simulink model "model_p3"  (R2020b)
settings: Solver=VariableStepAuto  StartTime=0.0  StopTime=10.0  RelTol=1e-3
settings Model: Creator=ADMIN  LastModifiedBy=ADMIN

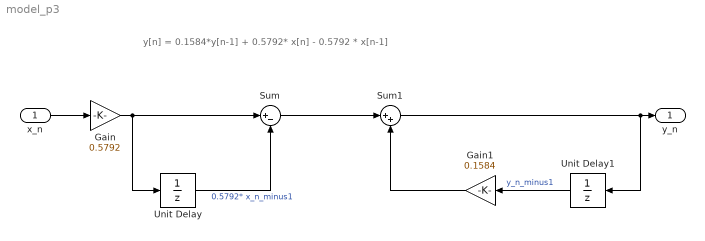
== system model_p3 ==
  note: y[n] = 0.1584*y[n-1] + 0.5792* x[n] - 0.5792 * x[n-1]
  x_n : Inport
  Gain : Gain  Gain=0.5792
  Gain1 : Gain  Gain=0.1584
  Sum : Sum  Inputs=|+-
  Sum1 : Sum  Inputs=|++
  Unit Delay : UnitDelay  SampleTime=-1  HasFrameUpgradeWarning=on
  Unit Delay1 : UnitDelay  SampleTime=-1  HasFrameUpgradeWarning=on
  y_n : Outport
  wires:
  x_n/1 -> Gain/1
  Gain/1 -> Sum/1, Unit Delay/1
  Unit Delay/1 -> Sum/2  "0.5792* x_n_minus1"
  Sum/1 -> Sum1/1
  Sum1/1 -> Unit Delay1/1, y_n/1
  Unit Delay1/1 -> Gain1/1  "y_n_minus1"
  Gain1/1 -> Sum1/2
